simulink model "white_noise_whistle4"  (Simulink 7.3)
settings: Solver=ode3  StartTime=0.0  StopTime=1  FixedStep=1/11025  MaxStep=1/11025  MinStep=1/11025  RelTol=1e-3
libraries: simulink x2, simulink_extras x1
settings Model: Creator=Hörnstein  LastModifiedBy=Hörnstein
settings SolverCC: InitialStep=1/11025
settings OptimizationCC: InitFltsAndDblsToZero=on
settings DebuggingCC: AlgebraicLoopMsg=none  SaveWithParameterizedLinksMsg=none  SignalResolutionControl=TryResolveAllWithWarning  MultiTaskDSMMsg=warning  MultiTaskCondExecSysMsg=none
settings RTWCC: IncludeERTFirstTime=on
settings GRTTargetCC: TargetFcnLib=ansi_tfl_tmw.mat

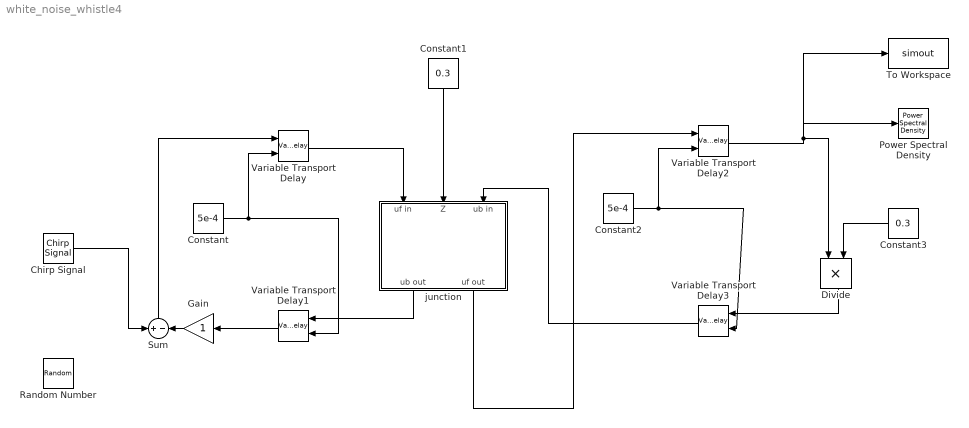
== system white_noise_whistle4 ==
  Chirp Signal : simulink/Sources/Chirp Signal  SystemSampleTime=-1  f1=0  T=1  f2=2000
  Constant : Constant  Value=5e-4  OutDataType=sfix(16)  OutScaling=2^0
  Constant1 : Constant  Value=0.3  OutDataType=sfix(16)  OutScaling=2^0
  Constant2 : Constant  Value=5e-4  OutDataType=sfix(16)  OutScaling=2^0
  Constant3 : Constant  Value=0.3  OutDataType=sfix(16)  OutScaling=2^0
  Divide : Product  Inputs=**  OutDataType=sfix(16)  OutScaling=2^-10
  Gain : Gain  ParameterDataType=sfix(16)  ParameterScaling=2^0  OutDataType=sfix(16)  OutScaling=2^0
  Power Spectral Density : simulink_extras/Additional Sinks/Power Spectral Density  SystemSampleTime=-1  npts=1102  fftpts=1102  HowOften=64  sampleT=1/11025
  Random Number : RandomNumber  SampleTime=0
  Sum : Sum  Inputs=+|-  OutDataType=sfix(16)  OutScaling=2^0
  To Workspace : ToWorkspace  VariableName=simout  SampleTime=-1  SaveFormat=Array
  Variable Transport Delay{,1..3} (4 alike) : VariableTransportDelay  VariableDelayType=Variable transport delay  MaximumDelay=10
  junction : Subsystem
  wires:
  Constant1/1 -> junction/2(Z)
  Sum/1 -> Variable Transport Delay/1
  Gain/1 -> Sum/2
  Chirp Signal/1 -> Sum/1
  junction/2(uf out) -> Variable Transport Delay2/1
  Variable Transport Delay/1 -> junction/1(uf in)
  junction/1(ub out) -> Variable Transport Delay1/1
  Variable Transport Delay1/1 -> Gain/1
  Constant/1 -> Variable Transport Delay1/2, Variable Transport Delay/2
  Variable Transport Delay3/1 -> junction/3(ub in)
  Constant2/1 -> Variable Transport Delay2/2, Variable Transport Delay3/2
  Variable Transport Delay2/1 -> To Workspace/1, Power Spectral Density/1, Divide/1
  Constant3/1 -> Divide/2
  Divide/1 -> Variable Transport Delay3/1

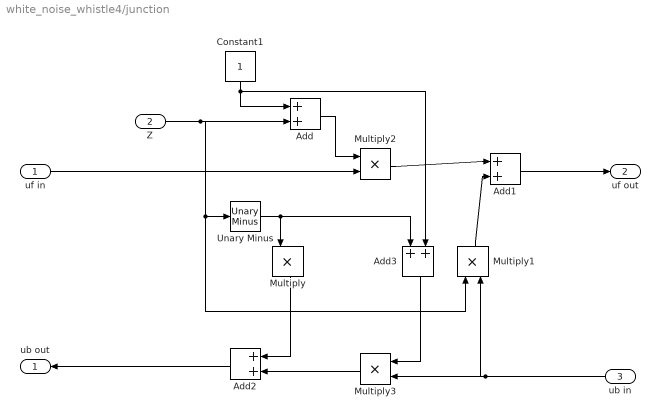
== system white_noise_whistle4/junction ==
  uf in : Inport  OutDataType=sfix(16)  OutScaling=2^0
  Z : Inport  Port=2  OutDataType=sfix(16)  OutScaling=2^0
  ub in : Inport  Port=3  OutDataType=sfix(16)  OutScaling=2^0
  Add{,1..3} (4 alike) : Sum  OutDataType=fixdt(1, 16)  OutScaling=2^-10
  Constant1 : Constant  OutDataType=sfix(16)  OutScaling=2^0
  Multiply{,1..3} (4 alike) : Product  Inputs=**  OutDataType=sfix(16)  OutScaling=2^-10
  Unary Minus : simulink/Math Operations/Unary Minus  DoSatur=off
  ub out : Outport  OutDataType=sfix(16)  OutScaling=2^0
  uf out : Outport  Port=2  OutDataType=sfix(16)  OutScaling=2^0
  wires:
  Add1/1 -> uf out/1
  Z/1 -> Add/2, Unary Minus/1, Multiply1/1
  Unary Minus/1 -> Multiply/1, Add3/1
  Constant1/1 -> Add/1, Add3/2
  Add/1 -> Multiply2/1
  Multiply2/1 -> Add1/1
  Multiply1/1 -> Add1/2
  Multiply/1 -> Add2/1
  Multiply3/1 -> Add2/2
  ub in/1 -> Multiply3/2, Multiply1/2
  Add3/1 -> Multiply3/1
  uf in/1 -> Multiply2/2
  Add2/1 -> ub out/1
